simulink model "m_heatbalance"  (R2020b)
settings: Solver=VariableStepAuto  StartTime=0.0  StopTime=Endtime  RelTol=1e-3
values from neighbouring files (symbols this model uses):
  C = pi*D^2/4    (= 0.196349540849)    [m_mbd_02_04.m]    (also in s_heatbalance.m = 4200)
  d0 = 20    [s_heatbalance.m]
  q_in = 1e-3    (= 0.001)    [m_mbd_02_04.m]    (also in s_heatbalance.m = 300)
  R = 500    [m_mbd_02_04.m]    (also in s_heatbalance.m = 0.1)
settings Model: Creator=005274  LastModifiedBy=005274

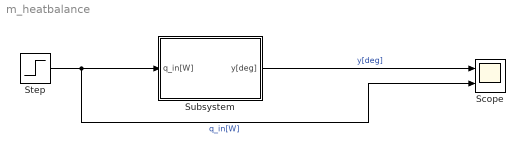
== system m_heatbalance ==
  Scope : Scope  NumInputPorts=2
  Step : Step  Time=100  After=q_in  SampleTime=0
  Subsystem : Subsystem
  wires:
  Step/1 -> Scope/2, Subsystem/1(q_in[W])  "q_in[W]"
  Subsystem/1(y[deg]) -> Scope/1  "y[deg]"

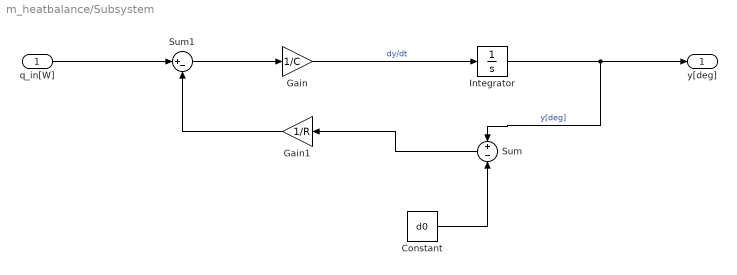
== system m_heatbalance/Subsystem ==
  q_in[W] : Inport
  Constant : Constant  Value=d0
  Gain : Gain  Gain=1/C
  Gain1 : Gain  Gain=1/R
  Integrator : Integrator  InitialCondition=d0
  Sum : Sum  Inputs=+-
  Sum1 : Sum  Inputs=|+-
  y[deg] : Outport
  wires:
  Gain/1 -> Integrator/1  "dy/dt"
  Gain1/1 -> Sum1/2
  Integrator/1 -> y[deg]/1, Sum/1  "y[deg]"
  Constant/1 -> Sum/2
  Sum/1 -> Gain1/1
  Sum1/1 -> Gain/1
  q_in[W]/1 -> Sum1/1
